simulink model "Care_Key_Max_Speed"  (R2022b)
settings: configuration reference "CommonModelConfiguration" (kept outside this file)
undefined symbols (not defined in the file): cc_param_214, cc_param_260
settings Model: Creator=rkallum  LastModifiedBy=othomso1
settings ConfigSetRef: SourceName=CommonModelConfiguration  SourceLocation=Base Workspace

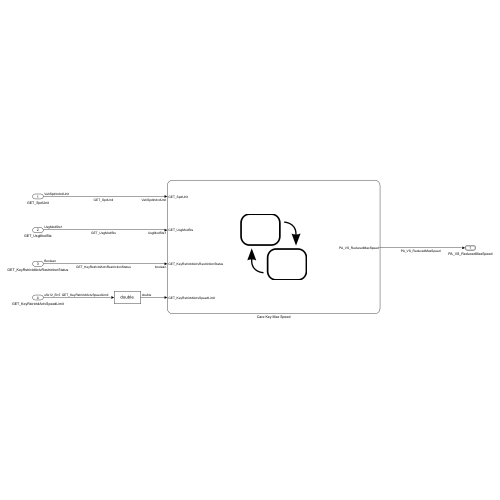
[thumbnail: Simulink's stored preview of the top-level diagram]
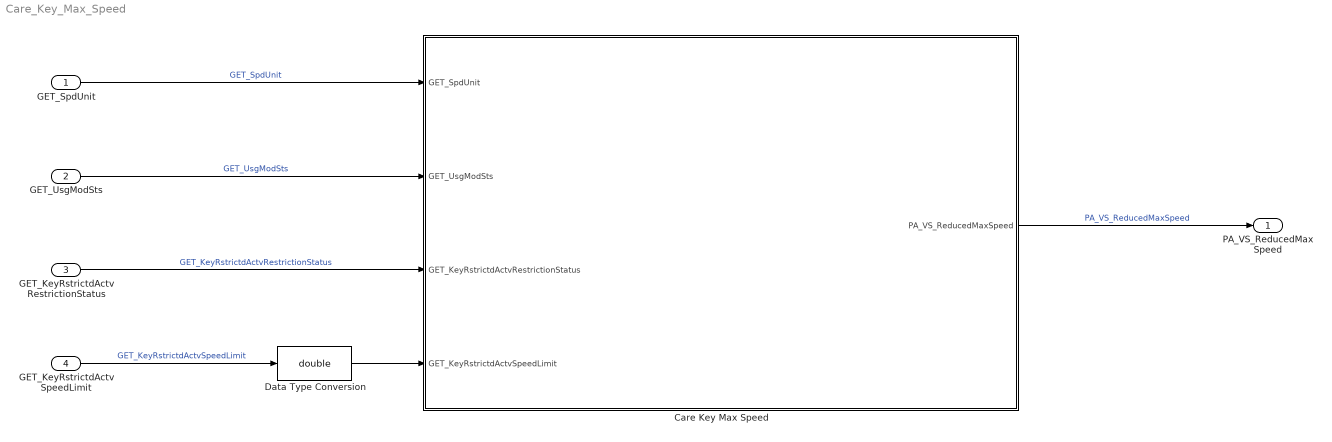
== system Care_Key_Max_Speed ==
  GET_SpdUnit : Inport  OutDataTypeStr=Enum: VehSpdIndcdUnit
  GET_UsgModSts : Inport  Port=2  OutDataTypeStr=Enum: UsgModSts1
  GET_KeyRstrictdActvRestrictionStatus : Inport  Port=3  OutDataTypeStr=Enum: Boolean
  GET_KeyRstrictdActvSpeedLimit : Inport  Port=4  OutDataTypeStr=Spd4
  Care Key Max Speed : Stateflow chart  TreatAsAtomicUnit=on
  Data Type Conversion : DataTypeConversion  OutDataTypeStr=double  SaturateOnIntegerOverflow=off  RndMeth=Floor
  PA_VS_ReducedMaxSpeed : Outport  OutDataTypeStr=Bus: PA_StatusAndDouble  VectorParamsAs1DForOutWhenUnconnected=off
  wires:
  GET_SpdUnit/1 -> Care Key Max Speed/1(GET_SpdUnit)  "GET_SpdUnit"
  Care Key Max Speed/1(PA_VS_ReducedMaxSpeed) -> PA_VS_ReducedMaxSpeed/1  "PA_VS_ReducedMaxSpeed"
  GET_UsgModSts/1 -> Care Key Max Speed/2(GET_UsgModSts)  "GET_UsgModSts"
  GET_KeyRstrictdActvRestrictionStatus/1 -> Care Key Max Speed/3(GET_KeyRstrictdActvRestrictionStatus)  "GET_KeyRstrictdActvRestrictionStatus"
  GET_KeyRstrictdActvSpeedLimit/1 -> Data Type Conversion/1  "GET_KeyRstrictdActvSpeedLimit"
  Data Type Conversion/1 -> Care Key Max Speed/4(GET_KeyRstrictdActvSpeedLimit)

== stateflow chart Care_Key_Max_Speed/Care Key Max Speed ==
  state CARCONFIG_INVALID
    entry: PA_VS_ReducedMaxSpeed.Status=E_CommonStatus.NotPresent;
    PA_VS_ReducedMaxSpeed.Value=0;
  state SYSTEM_OK
    state NOT_ACTIVE
      entry: PA_VS_ReducedMaxSpeed.Status=E_CommonStatus.Disabled;
      PA_VS_ReducedMaxSpeed.Value=0;
    state ACTIVE
      state ON
        entry: PA_VS_ReducedMaxSpeed.Status=E_CommonStatus.Available
        (default) -> (junction 124)
        ON -> (junction 124) [order 1]
        (junction 124) -> (junction 129) [order 1] : [GET_SpdUnit==VehSpdIndcdUnit.VehSpdIndcdUnit_Mph]
        (junction 124) -> (junction 127) [order 2] : {PA_VS_ReducedMaxSpeed.Value=GET_KeyRstrictdActvSpeedLimit*(36/10);}
        (junction 129) -> (junction 131) : {PA_VS_ReducedMaxSpeed.Value=GET_KeyRstrictdActvSpeedLimit*(1152/512);}
        (junction 131) -> (junction 127)
        (junction 127) -> (junction 134)
      state OFF
        entry: PA_VS_ReducedMaxSpeed.Status=E_CommonStatus.Disabled;
        PA_VS_ReducedMaxSpeed.Value=0;
      (default) -> (junction 161)
      (junction 161) -> OFF [order 2]
      (junction 161) -> ON [order 1] : [GET_KeyRstrictdActvRestrictionStatus == Boolean.Boolean_TRUE &&...
          | GET_KeyRstrictdActvSpeedLimit < 50 &&...
          | GET_KeyRstrictdActvSpeedLimit ~=0]
      OFF -> ON : %Restricted key detected
          | [GET_KeyRstrictdActvRestrictionStatus == Boolean.Boolean_TRUE &&...
          | GET_KeyRstrictdActvSpeedLimit < 50 &&...
          | GET_KeyRstrictdActvSpeedLimit ~=0]
      ON -> OFF [order 1] : %Restricted key not detected
          | [(GET_KeyRstrictdActvRestrictionStatus == Boolean.Boolean_FALSE) ||...
          | (GET_KeyRstrictdActvRestrictionStatus == Boolean.Boolean_TRUE &&...
          | (GET_KeyRstrictdActvSpeedLimit >= 50 ||...
          | GET_KeyRstrictdActvSpeedLimit == 0))]
    state isActive = activationCheck [function]
      (default) -> (junction 142)
      (junction 142) -> (junction 143) [order 1] : [GET_UsgModSts==UsgModSts1.UsgModSts1_UsgModDrvg ||...
          | GET_UsgModSts==UsgModSts1.UsgModSts1_UsgModActv]
      (junction 142) -> (junction 144) [order 2] : {isActive = false;}
      (junction 143) -> (junction 145) : {isActive = true;}
      (junction 145) -> (junction 144)
      (junction 144) -> (junction 146)
    (default) -> (junction 155)
    (junction 155) -> NOT_ACTIVE [order 1] : [~activationCheck()]
    (junction 155) -> (junction 158) [order 2]
    NOT_ACTIVE -> ACTIVE : [activationCheck()]
    ACTIVE -> NOT_ACTIVE : [~activationCheck()]
    (junction 158) -> ACTIVE
  (default) -> (junction 6)
  (junction 6) -> CARCONFIG_INVALID [order 2]
  (junction 6) -> SYSTEM_OK [order 1] : [cc_param_260>1 && cc_param_214==2]
  data: isActive function_output boolean; PA_VS_ReducedMaxSpeed output Bus: PA_StatusAndDouble; GET_SpdUnit input Enum: VehSpdIndcdUnit; cc_param_260 parameter double; cc_param_214 parameter double; GET_UsgModSts input Enum: UsgModSts1; GET_KeyRstrictdActvRestrictionStatus input Enum: Boolean; GET_KeyRstrictdActvSpeedLimit input double
